simulink model "threetanksimulink"  (R2017b)
settings: Solver=VariableStepAuto  StartTime=0.0  StopTime=10000.0  RelTol=1e-3
settings Model: Creator=root  LastModifiedBy=root

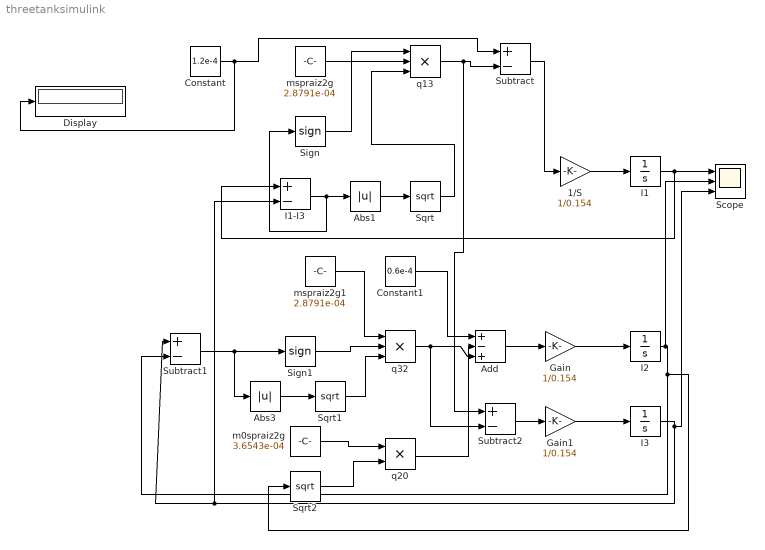
== system threetanksimulink ==
  1/S : Gain  Gain=1/0.154
  Abs1 : Abs
  Abs3 : Abs
  Add : Sum  Inputs=+-+
  Constant : Constant  Value=1.2e-4
  Constant1 : Constant  Value=0.6e-4
  Display : Display
  Gain : Gain  Gain=1/0.154
  Gain1 : Gain  Gain=1/0.154
  "I1 " : Integrator  InitialCondition=3.9353*10^(-2)
  I1-I3 : Sum  Inputs=+-
  I2 : Integrator  InitialCondition=7.4884*10^(-4)
  I3 : Integrator  InitialCondition=2.0051*10^(-2)
  Scope : Scope  NumInputPorts=3
  Sign : Signum
  Sign1 : Signum
  Sqrt : Sqrt  IntermediateResultsDataTypeStr=double  SaturateOnIntegerOverflow=on
  Sqrt1 : Sqrt  IntermediateResultsDataTypeStr=double  SaturateOnIntegerOverflow=on
  Sqrt2 : Sqrt  SaturateOnIntegerOverflow=on
  Subtract : Sum  Inputs=+-
  Subtract1 : Sum  Inputs=+-
  Subtract2 : Sum  Inputs=+-
  "m0spraiz2g " : Constant  Value=3.6543e-04
  mspraiz2g : Constant  Value=2.8791e-04
  mspraiz2g1 : Constant  Value=2.8791e-04
  "q13 " : Product  Inputs=3
  "q20 " : Product
  "q32 " : Product  Inputs=3
  wires:
  I3/1 -> Scope/3, Subtract1/1, I1-I3/2
  "I1 "/1 -> Scope/1, I1-I3/1
  I1-I3/1 -> Sign/1, Abs1/1
  Sqrt/1 -> "q13 "/3
  mspraiz2g/1 -> "q13 "/2
  Abs1/1 -> Sqrt/1
  Constant/1 -> Display/1, Subtract/1
  Subtract/1 -> 1/S/1
  1/S/1 -> "I1 "/1
  Gain/1 -> I2/1
  "q32 "/1 -> Subtract2/2, Add/3
  Add/1 -> Gain/1
  "q20 "/1 -> Add/2
  Constant1/1 -> Add/1
  mspraiz2g1/1 -> "q32 "/1
  Abs3/1 -> Sqrt1/1
  Sqrt1/1 -> "q32 "/3
  I2/1 -> Scope/2, Sqrt2/1, Subtract1/2
  Subtract1/1 -> Sign1/1, Abs3/1
  "m0spraiz2g "/1 -> "q20 "/1
  Sqrt2/1 -> "q20 "/2
  Gain1/1 -> I3/1
  Subtract2/1 -> Gain1/1
  "q13 "/1 -> Subtract2/1, Subtract/2
  Sign1/1 -> "q32 "/2
  Sign/1 -> "q13 "/1
